simulink model "environment_block_test"  (R2018b)
settings: Solver=VariableStepAuto  StartTime=0.0  StopTime=5000  RelTol=1e-3
undefined symbols (not defined in the file or in its folder): simParams
libraries: clock_lib x2, gravityGrad_Lib x1, atmoDrag_lib x1, solarPressure_lib x1, time_lib x1, Satellite_Dynamics_lib x1
settings Model: Creator=devantormey  LastModifiedBy=devantormey

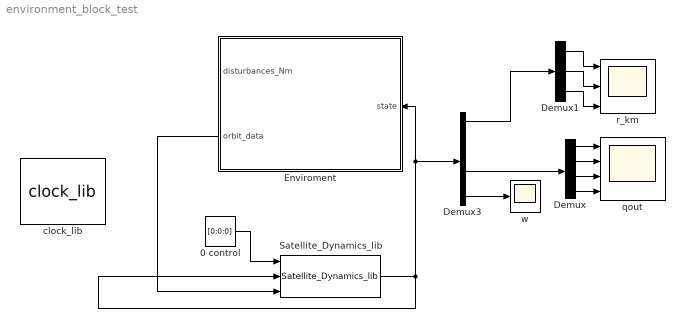
== system environment_block_test ==
  0 control : Constant  Value=[0;0;0]
  Demux : Demux
  Demux1 : Demux  Outputs=3
  Demux3 : Demux  Outputs=[3 3 4 3]
  Enviroment : Subsystem
  Satellite_Dynamics_lib : Satellite_Dynamics_lib/Satellite_Dynamics_lib  SystemSampleTime=-1
      link override Constant: Value=simParams.scParams.J
  clock_lib : clock_lib/clock_lib  SystemSampleTime=-1
  qout : Scope  NumInputPorts=4
  r_km : Scope  NumInputPorts=3
  w : Scope
  wires:
  Satellite_Dynamics_lib/1 -> Satellite_Dynamics_lib/2, Demux3/1, Enviroment/1(state)
  Enviroment/2(orbit_data) -> Satellite_Dynamics_lib/3
  0 control/1 -> Satellite_Dynamics_lib/1
  Demux1/3 -> r_km/3
  Demux/1 -> qout/1
  Demux3/4 -> w/1
  Demux/3 -> qout/3
  Demux3/3 -> Demux/1
  Demux3/1 -> Demux1/1
  Demux/2 -> qout/2
  Demux/4 -> qout/4
  Demux1/1 -> r_km/1
  Demux1/2 -> r_km/2

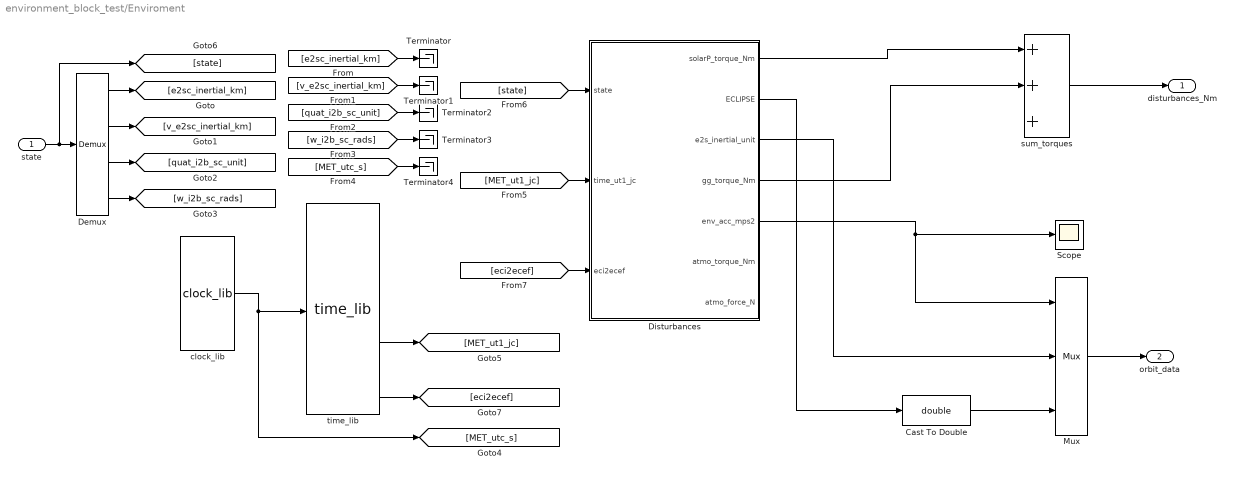
== system environment_block_test/Enviroment ==
  state : Inport
  Cast To Double : DataTypeConversion  OutDataTypeStr=double
  Demux : Demux  Outputs=[3 3 4 3]
  Disturbances : Subsystem
  Mux : Mux  Inputs=[3 3 1]
  Scope : Scope
  Terminator{,1..4} (5 alike) : Terminator
  clock_lib : clock_lib/clock_lib  SystemSampleTime=-1
  sum_torques : Sum  Inputs=+++
  "time_lib " : time_lib/time_lib    SystemSampleTime=-1
  disturbances_Nm : Outport
  orbit_data : Outport  Port=2
  wires:
  state/1 -> [state], Demux/1
  Demux/1 -> [e2sc_inertial_km]
  Demux/2 -> [v_e2sc_inertial_km]
  Demux/3 -> [quat_i2b_sc_unit]
  Demux/4 -> [w_i2b_sc_rads]
  clock_lib/1 -> "time_lib "/1, [MET_utc_s]
  "time_lib "/10 -> [MET_ut1_jc]
  "time_lib "/14 -> [eci2ecef]
  [eci2ecef] -> Disturbances/3(eci2ecef)
  Disturbances/4(gg_torque_Nm) -> sum_torques/2
  Disturbances/1(solarP_torque_Nm) -> sum_torques/1
  sum_torques/1 -> disturbances_Nm/1
  Disturbances/5(env_acc_mps2) -> Mux/1, Scope/1
  Disturbances/3(e2s_inertial_unit) -> Mux/2
  Mux/1 -> orbit_data/1
  [e2sc_inertial_km] -> Terminator/1
  [v_e2sc_inertial_km] -> Terminator1/1
  [quat_i2b_sc_unit] -> Terminator2/1
  [w_i2b_sc_rads] -> Terminator3/1
  [MET_utc_s] -> Terminator4/1
  [MET_ut1_jc] -> Disturbances/2(time_ut1_jc)
  [state] -> Disturbances/1(state)
  Cast To Double/1 -> Mux/3
  Disturbances/2(ECLIPSE) -> Cast To Double/1

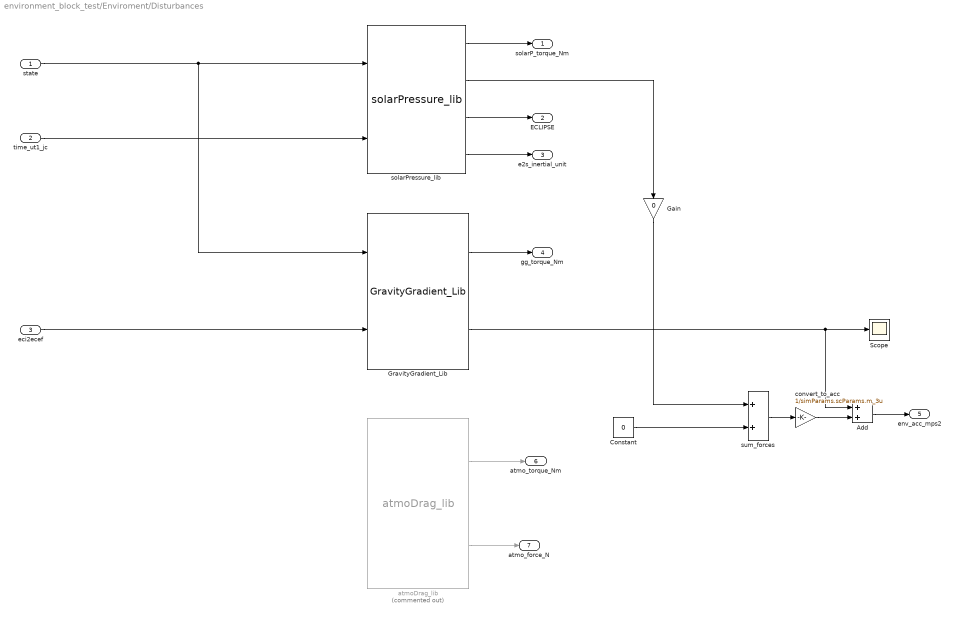
== system environment_block_test/Enviroment/Disturbances ==
  state : Inport
  time_ut1_jc : Inport  Port=2
  eci2ecef : Inport  Port=3
  Add : Sum
  Constant : Constant  Value=0
  Gain : Gain  Gain=0
  "GravityGradient_Lib " : gravityGrad_Lib/GravityGradient_Lib   SystemSampleTime=-1
  Scope : Scope
  atmoDrag_lib : atmoDrag_lib/atmoDrag_lib  Commented=on  SystemSampleTime=-1
  convert_to_acc : Gain  Gain=1/simParams.scParams.m_3u
  solarPressure_lib : solarPressure_lib/solarPressure_lib  SystemSampleTime=-1
  sum_forces : Sum
  solarP_torque_Nm : Outport
  ECLIPSE : Outport  Port=2
  e2s_inertial_unit : Outport  Port=3
  gg_torque_Nm : Outport  Port=4
  env_acc_mps2 : Outport  Port=5
  atmo_torque_Nm : Outport  Port=6
  atmo_force_N : Outport  Port=7
  wires:
  solarPressure_lib/3 -> ECLIPSE/1
  solarPressure_lib/1 -> solarP_torque_Nm/1
  solarPressure_lib/4 -> e2s_inertial_unit/1
  "GravityGradient_Lib "/1 -> gg_torque_Nm/1
  solarPressure_lib/2 -> Gain/1
  state/1 -> "GravityGradient_Lib "/1, solarPressure_lib/1
  time_ut1_jc/1 -> solarPressure_lib/2
  eci2ecef/1 -> "GravityGradient_Lib "/2
  sum_forces/1 -> convert_to_acc/1
  Add/1 -> env_acc_mps2/1
  convert_to_acc/1 -> Add/2
  "GravityGradient_Lib "/2 -> Scope/1, Add/1
  Constant/1 -> sum_forces/2
  atmoDrag_lib/1 -> atmo_torque_Nm/1
  atmoDrag_lib/2 -> atmo_force_N/1
  Gain/1 -> sum_forces/1
